simulink model "main_state_v3"  (R2021b)
settings: Solver=VariableStepAuto  StartTime=0.0  StopTime=10.0  RelTol=1e-3
settings Model: Creator=nose  LastModifiedBy=nose

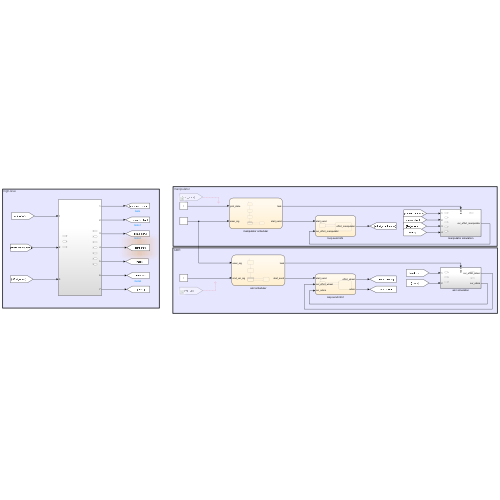
[thumbnail: Simulink's stored preview of the top-level diagram]
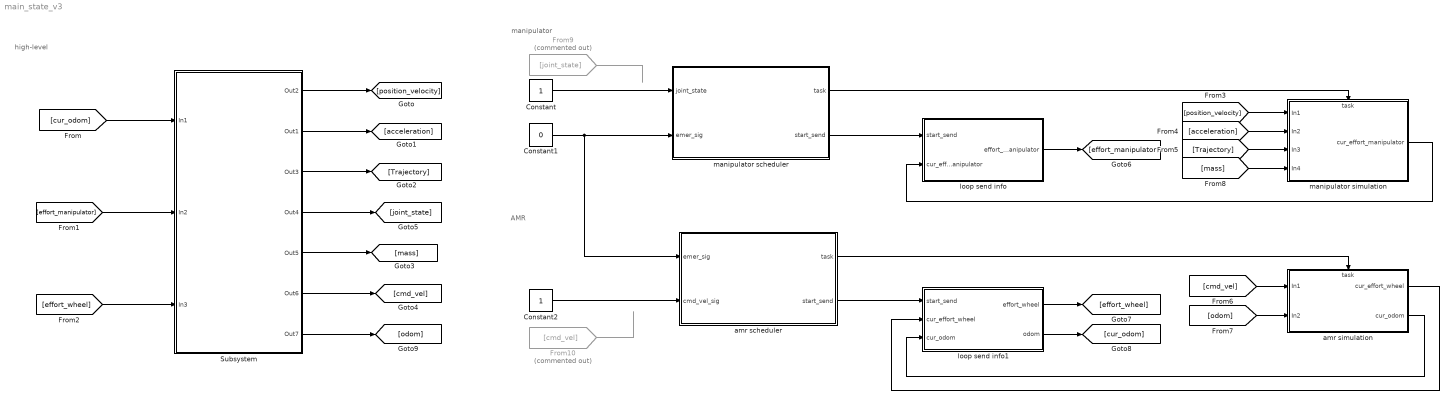
== system main_state_v3 ==
  note: high-level
  note: AMR
  note: manipulator
  Constant : Constant
  Constant1 : Constant  Value=0
  Constant2 : Constant
  From10 : From  Commented=on  GotoTag=cmd_vel
  From9 : From  Commented=on  GotoTag=joint_state
  Subsystem : Subsystem
  amr scheduler : Stateflow chart  TreatAsAtomicUnit=on
      settings: PortSchema="{\"entries\":[{\"content\":{\"sides\":[{\"content\":{\"connectorIds\":[\"In1\",\"In2\"]},\"type\":\"ConnectorPlacement.EquallySpacedRectSide\",\"uuid\":\"e14584fa-6c70-433d-b2da-38d1197773c6\"},{\"content\":{\"connectorIds\":[\"Out2\",\"Out1\"],\"side\":\"RIGHT\"},\"type\":\"ConnectorPlacement.EquallySpacedRectSide\",\"uuid\":\"c0129660-3601-4a2d-a8be-6a057e5db4e4\"},{\"content\":{\"connectorIds\":[],\"side\":\"TOP\"},\"type\":\"ConnectorPlacement.EquallySpacedRectSide\",\"uuid\":\"ad450ee9-aa73-4b1e-81ef-c89dc6269e7d\"}]},\"type\":\"ConnectorPlacement.EquallySpacedConnector\",\"uuid\":\"cc336b9e-cb49-4b3a-8aca-cb2cce9a2aaf\"}],\"packageUris\":[\"http://schema.mathworks.com/mf0/Connector/R2020b\"],\"version\":\"1.0\"}"
  amr simulation : Subsystem
      settings: PortSchema="{\"entries\":[{\"content\":{\"sides\":[{\"content\":{\"connectorIds\":[\"In1\",\"In2\"]},\"type\":\"ConnectorPlacement.EquallySpacedRectSide\",\"uuid\":\"e14584fa-6c70-433d-b2da-38d1197773c6\"},{\"content\":{\"connectorIds\":[\"Out1\",\"Out2\"],\"side\":\"RIGHT\"},\"type\":\"ConnectorPlacement.EquallySpacedRectSide\",\"uuid\":\"c0129660-3601-4a2d-a8be-6a057e5db4e4\"},{\"content\":{\"connectorIds\":[\"In3\"],\"side\":\"TOP\"},\"type\":\"ConnectorPlacement.EquallySpacedRectSide\",\"uuid\":\"ad450ee9-aa73-4b1e-81ef-c89dc6269e7d\"}]},\"type\":\"ConnectorPlacement.EquallySpacedConnector\",\"uuid\":\"cc336b9e-cb49-4b3a-8aca-cb2cce9a2aaf\"}],\"packageUris\":[\"http://schema.mathworks.com/mf0/Connector/R2020b\"],\"version\":\"1.0\"}"
  loop send info : Stateflow chart  TreatAsAtomicUnit=on
  loop send info1 : Stateflow chart  TreatAsAtomicUnit=on
  manipulator scheduler : Stateflow chart  TreatAsAtomicUnit=on
      settings: PortSchema="{\"entries\":[{\"content\":{\"sides\":[{\"content\":{\"connectorIds\":[\"In1\",\"In2\"]},\"type\":\"ConnectorPlacement.EquallySpacedRectSide\",\"uuid\":\"e14584fa-6c70-433d-b2da-38d1197773c6\"},{\"content\":{\"connectorIds\":[\"Out2\",\"Out1\"],\"side\":\"RIGHT\"},\"type\":\"ConnectorPlacement.EquallySpacedRectSide\",\"uuid\":\"c0129660-3601-4a2d-a8be-6a057e5db4e4\"},{\"content\":{\"connectorIds\":[],\"side\":\"TOP\"},\"type\":\"ConnectorPlacement.EquallySpacedRectSide\",\"uuid\":\"ad450ee9-aa73-4b1e-81ef-c89dc6269e7d\"}]},\"type\":\"ConnectorPlacement.EquallySpacedConnector\",\"uuid\":\"cc336b9e-cb49-4b3a-8aca-cb2cce9a2aaf\"}],\"packageUris\":[\"http://schema.mathworks.com/mf0/Connector/R2020b\"],\"version\":\"1.0\"}"
  manipulator simulation : Subsystem
      settings: PortSchema="{\"entries\":[{\"content\":{\"sides\":[{\"content\":{\"connectorIds\":[\"In1\",\"In2\",\"In3\",\"In4\"]},\"type\":\"ConnectorPlacement.EquallySpacedRectSide\",\"uuid\":\"80f1c3ab-f726-46f3-9980-68f35c05e058\"},{\"content\":{\"connectorIds\":[\"Out1\"],\"side\":\"RIGHT\"},\"type\":\"ConnectorPlacement.EquallySpacedRectSide\",\"uuid\":\"8613bb6a-65ca-45e7-9d44-92dca48eb7bb\"},{\"content\":{\"connectorIds\":[\"In5\"],\"side\":\"TOP\"},\"type\":\"ConnectorPlacement.EquallySpacedRectSide\",\"uuid\":\"e26f3b3a-06b4-4643-8203-7aff778e7067\"}]},\"type\":\"ConnectorPlacement.EquallySpacedConnector\",\"uuid\":\"cedcd8d2-6fb7-4e87-9ef3-c550760e1c47\"}],\"packageUris\":[\"http://schema.mathworks.com/mf0/Connector/R2020b\"],\"version\":\"1.0\"}"
  wires:
  manipulator scheduler/1(start_send) -> loop send info/1(start_send)
  Constant/1 -> manipulator scheduler/1(joint_state)
  Constant1/1 -> amr scheduler/1(emer_sig), manipulator scheduler/2(emer_sig)
  amr scheduler/1(start_send) -> loop send info1/1(start_send)
  Constant2/1 -> amr scheduler/2(cmd_vel_sig)
  Subsystem/1(Out2) -> [position_velocity]
  Subsystem/2(Out1) -> [acceleration]
  Subsystem/3(Out3) -> [Trajectory]
  Subsystem/4(Out4) -> [joint_state]
  Subsystem/5(Out5) -> [mass]
  Subsystem/6(Out6) -> [cmd_vel]
  loop send info/1(effort_manipulator) -> [effort_manipulator]
  loop send info1/1(effort_wheel) -> [effort_wheel]
  loop send info1/2(odom) -> [cur_odom]
  [cur_odom] -> Subsystem/1(In1)
  [effort_manipulator] -> Subsystem/2(In2)
  [effort_wheel] -> Subsystem/3(In3)
  [position_velocity] -> manipulator simulation/1(In1)
  [acceleration] -> manipulator simulation/2(In2)
  [Trajectory] -> manipulator simulation/3(In3)
  manipulator simulation/1(cur_effort_manipulator) -> loop send info/2(cur_effort_manipulator)
  [cmd_vel] -> amr simulation/1(In1)
  [odom] -> amr simulation/2(In2)
  amr simulation/1(cur_effort_wheel) -> loop send info1/2(cur_effort_wheel)
  amr simulation/2(cur_odom) -> loop send info1/3(cur_odom)
  Subsystem/7(Out7) -> [odom]
  [mass] -> manipulator simulation/4(In4)
  From9/1 -> ?
  manipulator scheduler/2(task) -> manipulator simulation/5(task)
  amr scheduler/2(task) -> amr simulation/3(task)
  From10/1 -> ?

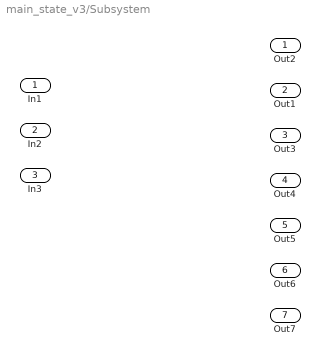
== system main_state_v3/Subsystem ==
  In1 : Inport
  In2 : Inport  Port=2
  In3 : Inport  Port=3
  Out2 : Outport
  Out1 : Outport  Port=2
  Out3 : Outport  Port=3
  Out4 : Outport  Port=4
  Out5 : Outport  Port=5
  Out6 : Outport  Port=6
  Out7 : Outport  Port=7

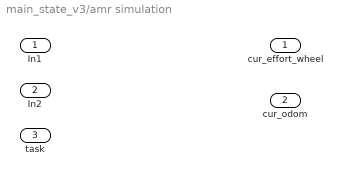
== system main_state_v3/amr simulation ==
  In1 : Inport
  In2 : Inport  Port=2
  task : Inport  Port=3
  cur_effort_wheel : Outport
  cur_odom : Outport  Port=2

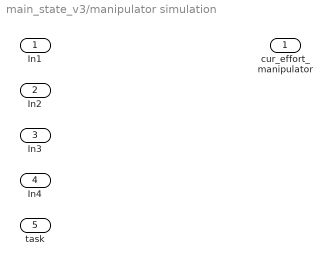
== system main_state_v3/manipulator simulation ==
  In1 : Inport
  In2 : Inport  Port=2
  In3 : Inport  Port=3
  In4 : Inport  Port=4
  task : Inport  Port=5
  cur_effort_manipulator : Outport

== stateflow chart main_state_v3/loop send info1 ==
  state send
    en:
    effort_wheel = cur_effort_wheel;
    odom = cur_odom;
    exit:
    effort_wheel = 0;
    odom = 0;
  state init
  (default) -> init
  init -> send : [start_send ==1]
  send -> init : after(100,msec)
  data: start_send input; effort_wheel output; odom output; cur_effort_wheel input; cur_odom input

== stateflow chart main_state_v3/loop send info ==
  state send
    en:
    effort_manipulator = cur_effort_manipulator;
    exit:
    effort_manipulator = 0;
  state init
  (default) -> init
  init -> send : [start_send ==1]
  send -> init : after(100,msec)
  data: effort_manipulator output; start_send input; cur_effort_manipulator input

== stateflow chart main_state_v3/manipulator scheduler ==
  state init
  state calibrate
  state home
  state working
    state init
      en:
      start_send = 0;
      task = 0;
    state move
      en:
      start_send = 1;
      task = 1;
    state pick
      en:
      start_send = 1;
      task = 2;
    state place
      en:
      start_send = 1;
      task = 3;
    (default) -> working.init
    move -> working.init
    working.init -> move [order 1] : [joint_state == 1]
    pick -> working.init
    working.init -> pick [order 2] : [joint_state == 2]
    place -> working.init
    working.init -> place [order 3] : [joint_state == 3]
  state emergency
  (default) -> init
  init -> calibrate
  calibrate -> home
  home -> working
  emergency -> working : [emer_sig == 0]
  working -> emergency : [emer_sig ==1]
  data: joint_state input; emer_sig input; start_send output; task output

== stateflow chart main_state_v3/amr scheduler ==
  state init
  state calibrate
  state working
    state init
      en:
      start_send = 0;
      task = 0;
    state move
      en:
      start_send = 1;
      task = 1;
    (default) -> working.init
    move -> working.init : [cmd_vel_sig == 0]
    working.init -> move : [cmd_vel_sig == 1]
  state emergency
  (default) -> init
  init -> calibrate
  calibrate -> working
  emergency -> working : [emer_sig == 0]
  working -> emergency : [emer_sig ==1]
  data: emer_sig input; start_send output; cmd_vel_sig input; task output
